simulink model "dcmPID_manual"  (R2020a)
settings: Solver=ode45  StartTime=0.0  StopTime=10.0  MaxStep=0.1  RelTol=1e-3  EnableMultiTasking=on
PreLoadFcn:
  | dcMotorParams
undefined symbols (not defined in the file): b, D, I, J, K, L, P, R
libraries: simulink x1
settings Model: Creator=deastman  LastModifiedBy=pawankumarf
settings DataIOCC: LimitDataPoints=on  SaveFormat=Array  SignalLoggingSaveFormat=ModelDataLogs  ReturnWorkspaceOutputs=off
settings OptimizationCC: ExpressionDepthLimit=2147483647  InitFltsAndDblsToZero=on  LifeSpan=inf
settings DebuggingCC: UnderspecifiedInitializationDetection=Classic  MergeDetectMultiDrivingBlocksExec=none  SolverPrmCheckMsg=warning  FcnCallInpInsideContextMsg=warning  StateNameClashWarn=warning  SFUnexpectedBacktrackingDiag=warning  SFNoUnconditionalDefaultTransitionDiag=warning  SFExecutionAtInitializationDiag=none  ArithmeticOperatorsInVariantConditions=warning
settings HardwareCC: ProdBitPerPointer=32  ProdBitPerSizeT=32  ProdBitPerPtrDiffT=32  ProdLargestAtomicFloat=None  ProdIntDivRoundTo=Undefined  ProdEndianess=Unspecified  ProdWordSize=32  ProdHWDeviceType=32-bit Generic
settings ModelReferenceCC: PropagateSignalLabelsOutOfModel=off
settings SFSimCC: SimUseLocalCustomCode=off  CustomCodeUndefinedFunction=UseInterfaceOnly
settings RTWCC: RTWUseLocalCustomCode=off
settings CodeAppCC: StateflowObjectComments=on
settings GRTTargetCC: TargetLangStandard=C89/C90 (ANSI)  CombineOutputUpdateFcns=off  GRTInterface=on
settings ConfigComp: CovMetricSettings=dw  CovHtmlReporting=on  CovSaveCumulativeToWorkspaceVar=on  CovSaveSingleToWorkspaceVar=on  CovExternalEMLEnable=off

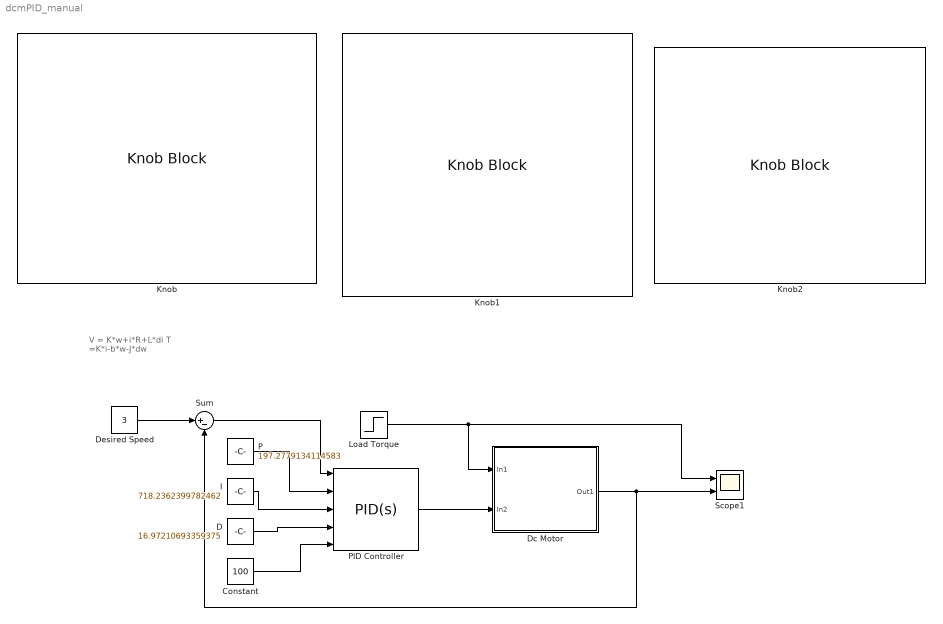
== system dcmPID_manual ==
  note: V = K*w+i*R+L*di
      | T =K*i-b*w-J*dw
  Constant : Constant  Value=100
  D : Constant  Value=16.97210693359375
  Dc Motor : Subsystem
      mask Display: image(imread('dcMotor.jpg'))
  Desired Speed : Constant  Value=3
  I : Constant  Value=718.2362399782462
  Knob : KnobBlock  ScaleMax=400
  Knob1 : KnobBlock  ScaleMax=1600
  Knob2 : KnobBlock  ScaleMax=30
  Load Torque : Step  Time=5  After=0.1  SampleTime=0
  P : Constant  Value=197.2779134114583
  PID Controller : simulink/Continuous/PID Controller  Controller=PID  Form=Parallel  TimeDomain=Continuous-time  UseExternalTs=off  SampleTime=-1  IntegratorMethod=Forward Euler  FilterMethod=Forward Euler  ControllerParametersSource=external  P=P  I=I  D=D  UseFilter=on  N=100  TunerSelectOption=Transfer Function Based (PID Tuner App)  InitialConditionSource=internal  InitialConditionForIntegrator=0  InitialConditionForFilter=0  DifferentiatorICPrevScaledInput=0  ExternalReset=none  TrackingMode=off  Kt=1  LimitOutput=off  UpperSaturationLimit=inf  LowerSaturationLimit=-inf  LinearizeAsGain=on  AntiWindupMode=none  Kb=1  POutMin=[]  POutMax=[]  IOutMin=[]  IOutMax=[]  DOutMin=[]  DOutMax=[]  NOutMin=[]  NOutMax=[]  SumOutMin=[]  SumOutMax=[]  SaturationOutMin=[]  SaturationOutMax=[]  PParamMin=[]  PParamMax=[]  IParamMin=[]  IParamMax=[]  DParamMin=[]  DParamMax=[]  NParamMin=[]  NParamMax=[]  KbParamMin=[]  KbParamMax=[]  KtParamMin=[]  KtParamMax=[]  KbOutMin=[]  KbOutMax=[]  KtOutMin=[]  KtOutMax=[]  IntegratorOutMin=[]  IntegratorOutMax=[]  FilterOutMin=[]  FilterOutMax=[]  SumI1OutMin=[]  SumI1OutMax=[]  SumI2OutMin=[]  SumI2OutMax=[]  SumI3OutMin=[]  SumI3OutMax=[]  SumI4OutMin=[]  SumI4OutMax=[]  SumDOutMin=[]  SumDOutMax=[]  DifferentiatorOutMin=[]  DifferentiatorOutMax=[]  FilterDiffOutCoefMin=[]  FilterDiffOutCoefMax=[]  ReciprocalOutMin=[]  ReciprocalOutMax=[]  SumDenOutMin=[]  SumDenOutMax=[]  SumNumOutMin=[]  SumNumOutMax=[]  DivideOutMin=[]  DivideOutMax=[]  UdiffTsProdOutMin=[]  UdiffTsProdOutMax=[]  NTsProdOutMin=[]  NTsProdOutMax=[]  UintegralTsProdOutMin=[]  UintegralTsProdOutMax=[]  UngainTsProdOutMin=[]  UngainTsProdOutMax=[]  IntegratorContinuousStateAttributes=''  IntegratorStateMustResolveToSignalObject=off  IntegratorRTWStateStorageClass=Auto  FilterContinuousStateAttributes=''  FilterStateMustResolveToSignalObject=off  FilterRTWStateStorageClass=Auto  ParallelPVariant=ExternalParameters  IdealPVariant=Disabled  IVariant=ExternalParameters  DVariant=ExternalParameters  IntegratorVariant=Continuous  SatVariant=Disabled  AWVariant=Passthrough  PCopyVariant=Disabled  TRVariant=Disabled  FdbkBlocksVariant=Forward  IdealPFdbkVariant=Disabled  SatFdbkVariant=Disabled  DerivativeFilterVariant=ContFilter  NVariant=ExternalParameters  NCopyVariant=Disabled  FilterICVariant=InternalICsFilter  IntegratorICVariant=InternalICs  ExternalResetVariant=Disabled  TRSumVariant=Passthrough  SumFdbkVariant=Disabled  SumVariant=Sum_PID  TsampFilterVariant=InternalTs  TsampNgainVariant=Passthrough  TsampIntegralVariant=Passthrough
  Scope1 : Scope  NumInputPorts=2
  Sum : Sum  Inputs=|+-
  wires:
  Dc Motor/1(Out1) -> Scope1/2, Sum/2
  Load Torque/1 -> Dc Motor/1(In1), Scope1/1
  Desired Speed/1 -> Sum/1
  Sum/1 -> PID Controller/1
  PID Controller/1 -> Dc Motor/2(In2)
  Constant/1 -> PID Controller/5
  P/1 -> PID Controller/2
  I/1 -> PID Controller/3
  D/1 -> PID Controller/4

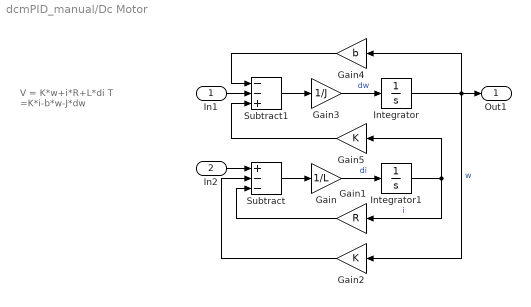
== system dcmPID_manual/Dc Motor ==
  note: V = K*w+i*R+L*di
      | T =K*i-b*w-J*dw
  In1 : Inport
  In2 : Inport  Port=2
  Gain : Gain  Gain=1/L
  Gain1 : Gain  Gain=R
  Gain2 : Gain  Gain=K
  Gain3 : Gain  Gain=1/J
  Gain4 : Gain  Gain=b
  Gain5 : Gain  Gain=K
  Integrator : Integrator
  Integrator1 : Integrator
  Subtract : Sum  Inputs=+--
  Subtract1 : Sum  Inputs=--+
  Out1 : Outport  VectorParamsAs1DForOutWhenUnconnected=off
  wires:
  Gain3/1 -> Integrator/1  "dw"
  Gain/1 -> Integrator1/1  "di"
  Integrator/1 -> Gain2/1, Gain4/1, Out1/1  "w"
  Integrator1/1 -> Gain1/1, Gain5/1  "i"
  Subtract/1 -> Gain/1
  Gain1/1 -> Subtract/3
  Gain2/1 -> Subtract/2
  Subtract1/1 -> Gain3/1
  Gain4/1 -> Subtract1/1
  Gain5/1 -> Subtract1/3
  In1/1 -> Subtract1/2
  In2/1 -> Subtract/1
